simulink model "sampleModel96"  (R2021b)
settings: Solver=VariableStepAuto  StartTime=0.0  StopTime=10.0  RelTol=1e-3
undefined symbols (not defined in the file or in its folder): Newton, Raphson
libraries: simulink x5, slpidlib x1
settings Model: Creator=user  LastModifiedBy=user

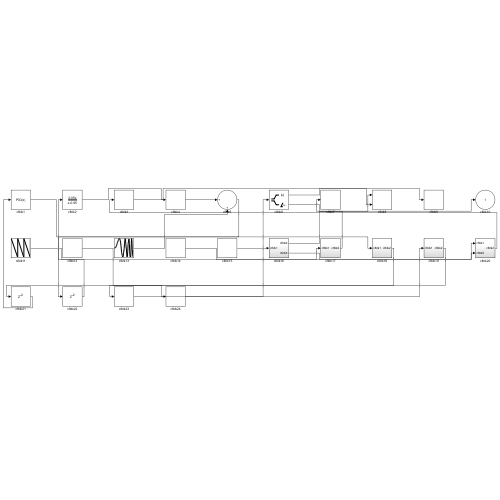
[thumbnail: Simulink's stored preview of the top-level diagram]
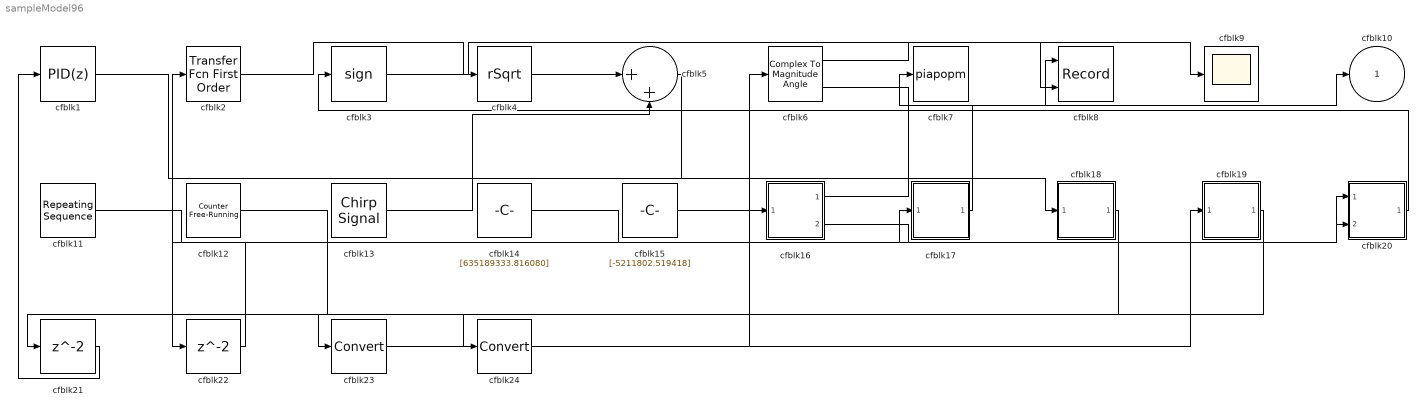
== system sampleModel96 ==
  cfblk1 : slpidlib/PID Controller  Controller=PID  Form=Parallel  TimeDomain=Discrete-time  UseExternalTs=off  SampleTime=1  IntegratorMethod=Forward Euler  FilterMethod=Forward Euler  ControllerParametersSource=internal  P=1  I=1  D=0  UseFilter=on  N=100  TunerSelectOption=Transfer Function Based (PID Tuner App)  InitialConditionSource=internal  InitialConditionForIntegrator=0  InitialConditionForFilter=0  DifferentiatorICPrevScaledInput=0  ExternalReset=none  TrackingMode=off  Kt=1  LimitOutput=off  SatLimitsSource=internal  UpperSaturationLimit=inf  LowerSaturationLimit=-inf  LinearizeAsGain=off  AntiWindupMode=none  Kb=1  POutMin=[]  POutMax=[]  IOutMin=[]  IOutMax=[]  DOutMin=[]  DOutMax=[]  NOutMin=[]  NOutMax=[]  SumOutMin=[]  SumOutMax=[]  SaturationOutMin=[]  SaturationOutMax=[]  PParamMin=[]  PParamMax=[]  IParamMin=[]  IParamMax=[]  DParamMin=[]  DParamMax=[]  NParamMin=[]  NParamMax=[]  KbParamMin=[]  KbParamMax=[]  KtParamMin=[]  KtParamMax=[]  KbOutMin=[]  KbOutMax=[]  KtOutMin=[]  KtOutMax=[]  IntegratorOutMin=[]  IntegratorOutMax=[]  FilterOutMin=[]  FilterOutMax=[]  SumI1OutMin=[]  SumI1OutMax=[]  SumI2OutMin=[]  SumI2OutMax=[]  SumI3OutMin=[]  SumI3OutMax=[]  SumI4OutMin=[]  SumI4OutMax=[]  SumDOutMin=[]  SumDOutMax=[]  DifferentiatorOutMin=[]  DifferentiatorOutMax=[]  FilterDiffOutCoefMin=[]  FilterDiffOutCoefMax=[]  ReciprocalOutMin=[]  ReciprocalOutMax=[]  SumDenOutMin=[]  SumDenOutMax=[]  SumNumOutMin=[]  SumNumOutMax=[]  DivideOutMin=[]  DivideOutMax=[]  UdiffTsProdOutMin=[]  UdiffTsProdOutMax=[]  NTsProdOutMin=[]  NTsProdOutMax=[]  UintegralTsProdOutMin=[]  UintegralTsProdOutMax=[]  UngainTsProdOutMin=[]  UngainTsProdOutMax=[]  IntegratorContinuousStateAttributes=''  IntegratorStateMustResolveToSignalObject=off  IntegratorRTWStateStorageClass=Auto  FilterContinuousStateAttributes=''  FilterStateMustResolveToSignalObject=off  FilterRTWStateStorageClass=Auto  ParallelPVariant=InternalParameters  IdealPVariant=Disabled  IVariant=InternalParameters  DVariant=InternalParameters  IntegratorVariant=Discrete  SatVariant=Disabled  AWVariant=Passthrough  PCopyVariant=Disabled  TRVariant=Disabled  FdbkBlocksVariant=Forward  IdealPFdbkVariant=Disabled  SatFdbkVariant=Disabled  DerivativeFilterVariant=ForwardEulerFilter  NVariant=InternalParameters  NCopyVariant=Disabled  FilterICVariant=InternalICsFilter  IntegratorICVariant=InternalICs  ExternalResetVariant=Disabled  TRSumVariant=Passthrough  SumFdbkVariant=Disabled  SumVariant=Sum_PID  TsampFilterVariant=InternalTs  TsampNgainVariant=Passthrough  TsampIntegralVariant=Passthrough  ExternalSaturationOutDataTypeStr=Inherit: Same as second input
  cfblk11 : simulink/Sources/Repeating Sequence  rep_seq_t=[0 2]  rep_seq_y=[993583180.391586, -379827873.670717]
  cfblk12 : simulink/Sources/Counter Free-Running  NumBits=[17.000000]  tsamp=-1
  cfblk13 : simulink/Sources/Chirp Signal  f1=[-589694791.899771]  T=[721164078.337193]  f2=[-743229759.537158]
  cfblk14 : Constant  Value=[635189333.816080]  SampleTime=1
  cfblk15 : Constant  Value=[-5211802.519418]  SampleTime=1
  cfblk16 : Subsystem
  cfblk17 : Subsystem
  cfblk18 : Subsystem
  cfblk19 : Subsystem
  cfblk2 : simulink/Discrete/Transfer Fcn First Order  PoleZ=0.95  ICPrevOutput=0.0  DoSatur=off
  cfblk20 : Subsystem
  cfblk21 : Delay  SampleTime=1
  cfblk22 : Delay  SampleTime=1
  cfblk23 : DataTypeConversion
  cfblk24 : DataTypeConversion
  cfblk3 : Signum
  cfblk4 : Sqrt  Operator=rSqrt  AlgorithmType=Newton-Raphson  SaturateOnIntegerOverflow=on
  cfblk5 : Sum  Inputs=|++
  cfblk6 : ComplexToMagnitudeAngle
  cfblk7 : ToWorkspace  VariableName=piapopm  SaveFormat=Timeseries  SampleTime=-1
  cfblk8 : Record  FileSettingsInternal="{\"entries\":[{\"content\":{\"excelSettings\":{\"content\":{},\"type\":\"Streamout.ExcelSettings\"}},\"type\":\"Streamout.FileSettingStorage\",\"uuid\":\"82a40183-930c-4ae2-b3b4-1305f3054bea\"}],\"packageUris\":[\"http://schema.mathworks.com/mf0/streamout_blocks/R2020a\"],\"version\":\"1.0\"}"  Layout=[1 1]  SignalsInternal="{\"entries\":[{\"content\":{\"signals\":[{\"content\":{\"blockPath\":[\"sampleModel96/cfblk8\"],\"channel\":[],\"dimensions\":[1],\"domain\":\"sampleModel96/cfblk8\",\"lineColor\":\"#a2142f\",\"plots\":[1],\"port\":1,\"sid\":[\"\"],\"signalID\":3405,\"signalName\":\"cfblk16:1\"},\"type\":\"RecordBlkView.Signal\",\"uuid\":\"b0fe5bac-beb1-4eda-9463-7d8108459b01\"},{\"content\":{\"blockPath\":[\"sampleModel96/cfblk8\"],\"channel\":[],\"dimensions\":[1],\"domain\":\"sampleModel96/cfblk8\",\"lineColor\":\"#139fff\",\"plots\":[1],\"port\":2,\"sid\":[\"\"],\"signalID\":3409,\"signalName\":\"cfblk3\"},\"type\":\"RecordBlkView.Signal\",\"uuid\":\"a879d078-84ac-459f-880d-d127f3ea6a9e\"}]},\"type\":\"RecordBlkView.InputSignals\",\"uuid\":\"0b755a0b-f5d3-4291-827d-a8148995142c\"}],\"packageUris\":[\"http://schema.mathworks.com/mf0/streamout_blocks/R2020a\"],\"version\":\"1.0\"}"  VisualizationBindings="{\"xyplotplugin\":{\"info\":[{\"series\":[{\"bindingParametersList\":[{\"parameter\":\"X-Axis\",\"signalID\":3405,\"signalName\":\"cfblk16:1\"},{\"parameter\":\"Y-Axis\",\"signalID\":3409,\"signalName\":\"cfblk3\"}],\"seriesID\":43629}],\"subplotID\":1}]}}"  CompatibilityTag=XY
  cfblk9 : Scope
  cfblk10 : Outport
  wires:
  cfblk6/1 -> cfblk9/1
  cfblk20/1(cfblk2) -> cfblk3/1
  cfblk16/1(cfblk2) -> cfblk8/1
  cfblk11/1 -> cfblk17/1(cfblk1)
  cfblk17/1(cfblk2) -> cfblk7/1
  cfblk6/2 -> cfblk10/1
  cfblk4/1 -> cfblk5/1
  cfblk15/1 -> cfblk16/1(cfblk1)
  cfblk1/1 -> cfblk18/1(cfblk1)
  cfblk16/2(cfblk5) -> cfblk20/1(cfblk1)
  cfblk13/1 -> cfblk5/2
  cfblk3/1 -> cfblk8/2
  cfblk14/1 -> cfblk20/2(cfblk5)
  cfblk2/1 -> cfblk4/1
  cfblk18/1(cfblk2) -> cfblk21/1
  cfblk21/1 -> cfblk1/1
  cfblk5/1 -> cfblk22/1
  cfblk22/1 -> cfblk2/1
  cfblk19/1(cfblk2) -> cfblk23/1
  cfblk23/1 -> cfblk6/1
  cfblk12/1 -> cfblk24/1
  cfblk24/1 -> cfblk19/1(cfblk1)

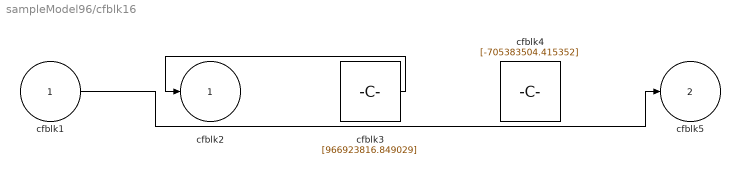
== system sampleModel96/cfblk16 ==
  cfblk1 : Inport
  cfblk3 : Constant  Value=[966923816.849029]  SampleTime=1
  cfblk4 : Constant  Value=[-705383504.415352]  SampleTime=1
  cfblk2 : Outport
  cfblk5 : Outport  Port=2
  wires:
  cfblk3/1 -> cfblk2/1
  cfblk1/1 -> cfblk5/1

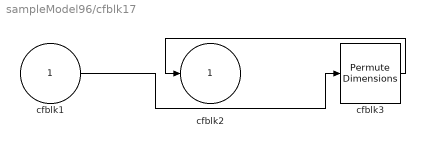
== system sampleModel96/cfblk17 ==
  cfblk1 : Inport
  cfblk3 : PermuteDimensions
  cfblk2 : Outport
  wires:
  cfblk3/1 -> cfblk2/1
  cfblk1/1 -> cfblk3/1

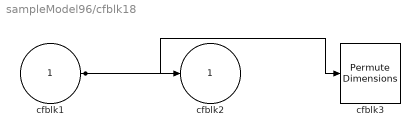
== system sampleModel96/cfblk18 ==
  cfblk1 : Inport
  cfblk3 : PermuteDimensions
  cfblk2 : Outport
  wires:
  cfblk1/1 -> cfblk2/1, cfblk3/1

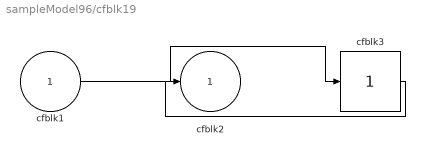
== system sampleModel96/cfblk19 ==
  cfblk1 : Inport
  cfblk3 : simulink/Math Operations/Slider Gain  gain=1  low=0  high=2
  cfblk2 : Outport
  wires:
  cfblk1/1 -> cfblk3/1
  cfblk3/1 -> cfblk2/1

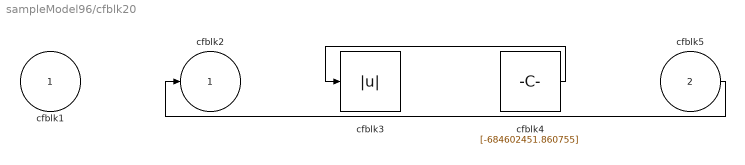
== system sampleModel96/cfblk20 ==
  cfblk1 : Inport
  cfblk5 : Inport  Port=2
  cfblk3 : Abs
  cfblk4 : Constant  Value=[-684602451.860755]  SampleTime=1
  cfblk2 : Outport
  wires:
  cfblk4/1 -> cfblk3/1
  cfblk5/1 -> cfblk2/1
